simulink model "Lab1_A (1)"  (R2020b)
settings: Solver=VariableStepAuto  StartTime=0.0  StopTime=10.0  RelTol=1e-3
undefined symbols (not defined in the file or in its folder): c, ic, l
settings Model: Creator=georg  LastModifiedBy=georg

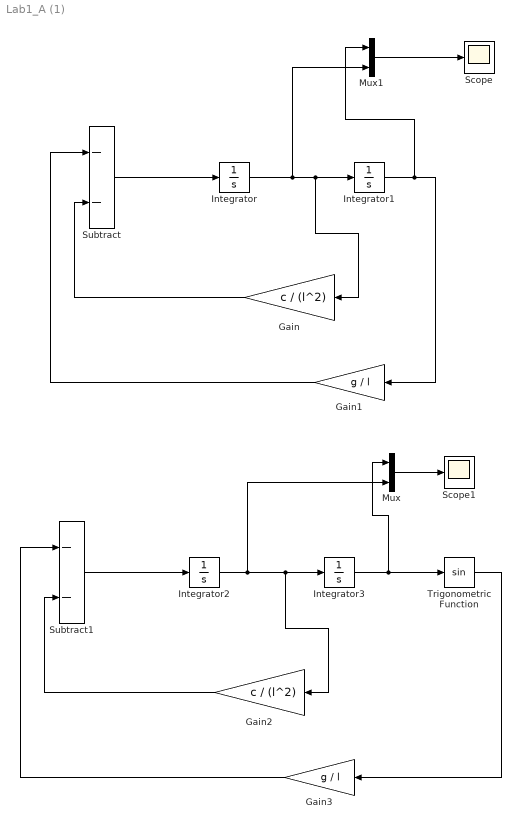
== system Lab1_A (1) ==
  Gain : Gain  Gain=c / (l^2)
  Gain1 : Gain  Gain=g / l
  Gain2 : Gain  Gain=c / (l^2)
  Gain3 : Gain  Gain=g / l
  Integrator : Integrator  InitialCondition=ic(2)
  Integrator1 : Integrator  InitialCondition=ic(1)
  Integrator2 : Integrator  InitialCondition=ic(2)
  Integrator3 : Integrator  InitialCondition=ic(1)
  Mux : Mux  Inputs=2
  Mux1 : Mux  Inputs=2
  Scope : Scope
  Scope1 : Scope
  Subtract : Sum  Inputs=--
  Subtract1 : Sum  Inputs=--
  Trigonometric Function : Trigonometry
  wires:
  Subtract/1 -> Integrator/1
  Integrator/1 -> Mux1/2, Gain/1, Integrator1/1
  Integrator1/1 -> Mux1/1, Gain1/1
  Gain/1 -> Subtract/2
  Gain1/1 -> Subtract/1
  Integrator2/1 -> Mux/2, Gain2/1, Integrator3/1
  Gain3/1 -> Subtract1/1
  Integrator3/1 -> Mux/1, Trigonometric Function/1
  Subtract1/1 -> Integrator2/1
  Gain2/1 -> Subtract1/2
  Trigonometric Function/1 -> Gain3/1
  Mux/1 -> Scope1/1
  Mux1/1 -> Scope/1
